simulink library "TEsim_utils"  (R2014a)
settings: Solver=ode45  StartTime=0.0  StopTime=10.0  RelTol=1e-3
settings Model: Creator=rnc4  LastModifiedBy=rnc4

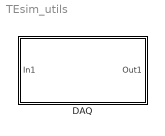
== system TEsim_utils ==
  DAQ : Subsystem  mask{time_slot_dur_ms=10, time_slot_num=0}
      mask prompts: time_slot_dur_ms "Time slot duration (ms):"; time_slot_num "Time slot"
      mask Display:
      | port_label('input',1,'x(t)')
      | port_label('output',1,'x[k]')
      | 
      | text(.5,.5,'DAQ: x(t) \rightarrow x[k]','hor','center','texmode','on')

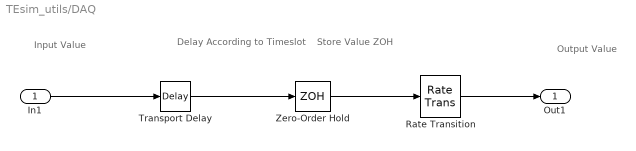
== system TEsim_utils/DAQ ==
  note: Delay According
      | to Timeslot
  note: Input Value
  note: Store Value
      | ZOH
  note: Output Value
  In1 : Inport
  Rate Transition : RateTransition  OutPortSampleTime=time_slot_dur_ms/1000
  Transport Delay : TransportDelay  DelayTime=time_slot_dur_ms/1000*time_slot_num
  Zero-Order Hold : ZeroOrderHold  SampleTime=time_slot_dur_ms/1000
  Out1 : Outport
  wires:
  In1/1 -> Transport Delay/1
  Transport Delay/1 -> Zero-Order Hold/1
  Zero-Order Hold/1 -> Rate Transition/1
  Rate Transition/1 -> Out1/1
